simulink model "second_order_case1"  (R2023a)
settings: Solver=VariableStepAuto  StartTime=0.0  StopTime=10.0  MaxStep=1e-3
values from neighbouring files (symbols this model uses):
  wn = 1/(R1*C1)    (= 1000)    [Case1_script.m]
  zeta = ((R1*C1)+(R1*C2)+(R2*C2))/(2*wn*(R1*R2*C1*C2))    (= 1.5)    [Case1_script.m]
settings Model: Creator=mazen  LastModifiedBy=mazen

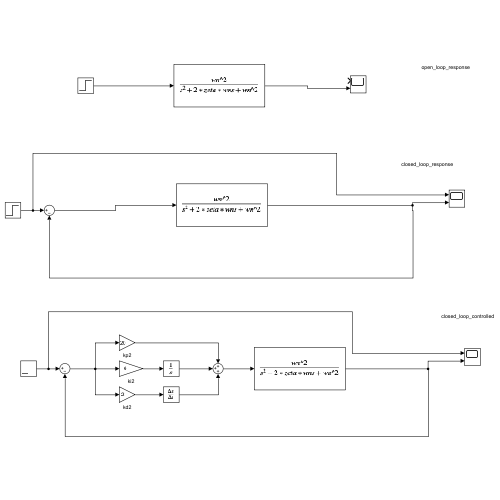
[thumbnail: Simulink's stored preview of the top-level diagram]
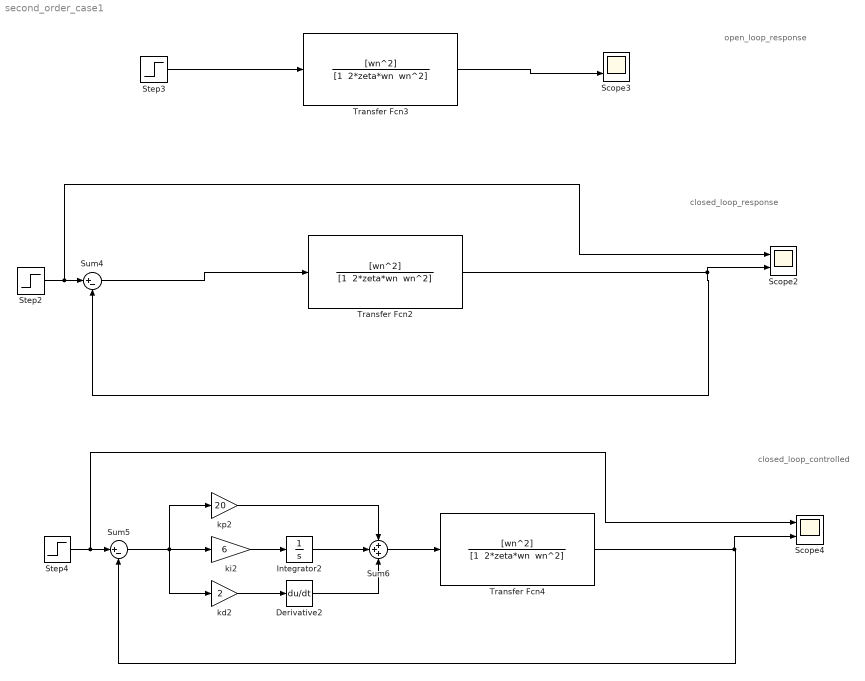
== system second_order_case1 ==
  note: closed_loop_controlled
  note: closed_loop_response
  note: open_loop_response
  Derivative2 : Derivative
  Integrator2 : Integrator
  Scope2 : Scope  NumInputPorts=2
  Scope3 : Scope  NumInputPorts=2
  Scope4 : Scope  NumInputPorts=2
  Step2 : Step  SampleTime=0
  Step3 : Step  SampleTime=0
  Step4 : Step  SampleTime=0
  Sum4 : Sum  Inputs=|+-
  Sum5 : Sum  Inputs=|+-
  Sum6 : Sum  Inputs=+++
  Transfer Fcn2 : TransferFcn  Numerator=[wn^2]  Denominator="[1  2*zeta*wn  wn^2]"
  Transfer Fcn3 : TransferFcn  Numerator=[wn^2]  Denominator="[1  2*zeta*wn  wn^2]"
  Transfer Fcn4 : TransferFcn  Numerator=[wn^2]  Denominator="[1  2*zeta*wn  wn^2]"
  kd2 : Gain  Gain=2
  ki2 : Gain  Gain=6
  kp2 : Gain  Gain=20
  wires:
  Transfer Fcn2/1 -> Sum4/2, Scope2/2
  Step2/1 -> Scope2/1, Sum4/1
  Sum4/1 -> Transfer Fcn2/1
  Step3/1 -> Transfer Fcn3/1
  Transfer Fcn3/1 -> Scope3/2
  Sum6/1 -> Transfer Fcn4/1
  Sum5/1 -> kp2/1, ki2/1, kd2/1
  kp2/1 -> Sum6/1
  Derivative2/1 -> Sum6/3
  Integrator2/1 -> Sum6/2
  ki2/1 -> Integrator2/1
  kd2/1 -> Derivative2/1
  Step4/1 -> Sum5/1, Scope4/1
  Transfer Fcn4/1 -> Scope4/2, Sum5/2
